simulink model "sixdof"  (R2023a)
settings: Solver=FixedStepAuto  StartTime=0.0  StopTime=5000  FixedStep=0.01  RelTol=1e-3  EnableMultiTasking=on
InitFcn:
  | fox_loadvariables_new
model workspace (MAT data in the model file):
  waypoints = [0  0  20; 1000  0  20; 1000  1000  20; -1000  1000  20; 0  0  20]
values from neighbouring files (symbols this model uses):
  Apolar = 0.038    [fox_loadvariables_new.m]
  CD0 = 0.0191    [fox_loadvariables_new.m]
  chord = chord*0.3048    (= 0.3048)    [fox_loadvariables_new.m]
  CL0 = 3*0.076    (= 0.228)    [fox_loadvariables_new.m]
  CLa = 5.097    [fox_loadvariables_new.m]
  CLa_dot = 1.93    [fox_loadvariables_new.m]
  Clb = -0.0598    [fox_loadvariables_new.m]
  ClDa = 0.265    [fox_loadvariables_new.m]
  CLDe = 0.738    [fox_loadvariables_new.m]
  ClDr = 0.0064    [fox_loadvariables_new.m]
  Clp = -0.363    [fox_loadvariables_new.m]
  CLq = 6.03    [fox_loadvariables_new.m]
  Clr = 0.0886    [fox_loadvariables_new.m]
  Cm0 = 0.107    [fox_loadvariables_new.m]
  Cma = -2.051    [fox_loadvariables_new.m]
  Cma_dot = -5.286    [fox_loadvariables_new.m]
  CmDe = -2.021    [fox_loadvariables_new.m]
  Cmq = -16.52    [fox_loadvariables_new.m]
  Cnb = 0.0562    [fox_loadvariables_new.m]
  CnDa = -0.0296    [fox_loadvariables_new.m]
  CnDr = -0.0377    [fox_loadvariables_new.m]
  Cnp = -0.0407    [fox_loadvariables_new.m]
  Cnr = -0.0439    [fox_loadvariables_new.m]
  CYb = -0.204    [fox_loadvariables_new.m]
  CYDr = 0.112    [fox_loadvariables_new.m]
  Euler_0 = [0; 0; 180]'*pi/180    [fox_loadvariables_new.m]
  ISA_g = 9.815    [fox_loadvariables_new.m]
  ISA_hmax = 2000    [fox_loadvariables_new.m]
  ISA_lapse = .0065    (= 0.0065)    [fox_loadvariables_new.m]
  ISA_P0 = 101325    [fox_loadvariables_new.m]
  ISA_R = 287    [fox_loadvariables_new.m]
  ISA_rho0 = 1.225    [fox_loadvariables_new.m]
  ISA_T0 = 289    [fox_loadvariables_new.m]
  Ixx = Ixx*1.355817949    (= 0.363359210332)    [fox_loadvariables_new.m]
  Iyy = Iyy*1.355817949    (= 0.86772348736)    [fox_loadvariables_new.m]
  Izz = Izz*1.355817949    (= 1.19854306692)    [fox_loadvariables_new.m]
  mass = mass*0.45359237    (= 9.0718474)    [fox_loadvariables_new.m]
  Pos_0 = [0; 0; 100.]    [fox_loadvariables_new.m]
  PQR_0 = [0; 0; 0]'    [fox_loadvariables_new.m]
  span = span*0.3048    (= 2.4384)    [fox_loadvariables_new.m]
  Vb_0 = [85.; 0; 0]'*0.3048    [fox_loadvariables_new.m]
undefined symbols (not defined in the file or in its folder): YPGwind
libraries: simulink x5, slpidlib x5, sharedtransform x1, uavutilslib x1, uavalgslib x1
(part 1 of 2)
settings Model: Creator=anouck  LastModifiedBy=terry
settings SolverCC: AlgebraicLoopSolver=TrustRegion  EnableFixedStepZeroCrossing=on
settings DataIOCC: LimitDataPoints=on  SaveFormat=Array  SignalLoggingSaveFormat=ModelDataLogs  ReturnWorkspaceOutputs=off  SignalLoggingName=sigsOut
settings OptimizationCC: ExpressionDepthLimit=2147483647  LifeSpan=inf
settings DebuggingCC: SaveWithParameterizedLinksMsg=none  UnderspecifiedInitializationDetection=Classic  MergeDetectMultiDrivingBlocksExec=none  SignalResolutionControl=TryResolveAllWithWarning  MultiTaskDSMMsg=warning  MultiTaskCondExecSysMsg=none  FcnCallInpInsideContextMsg=warning  UnconnectedInputMsg=warning  UnconnectedOutputMsg=warning  UnconnectedLineMsg=warning  StateNameClashWarn=warning  SFUnexpectedBacktrackingDiag=warning  SFNoUnconditionalDefaultTransitionDiag=warning  SFExecutionAtInitializationDiag=none  ArithmeticOperatorsInVariantConditions=warning
settings HardwareCC: ProdBitPerPointer=32  ProdBitPerSizeT=32  ProdBitPerPtrDiffT=32  ProdLargestAtomicFloat=None  ProdIntDivRoundTo=Undefined  ProdEndianess=Unspecified  ProdWordSize=32  ProdHWDeviceType=32-bit Generic  TargetBitPerPointer=64  TargetBitPerSizeT=64  TargetBitPerPtrDiffT=64  TargetLongLongMode=on  TargetIntDivRoundTo=Zero  TargetEndianess=LittleEndian  TargetWordSize=64  TargetHWDeviceType=MATLAB Host  ProdEqTarget=off
settings ModelReferenceCC: PropagateSignalLabelsOutOfModel=off
settings SFSimCC: SimUseLocalCustomCode=off  CustomCodeUndefinedFunction=UseInterfaceOnly
settings RTWCC: RTWUseLocalCustomCode=off
settings CodeAppCC: StateflowObjectComments=on
settings GRTTargetCC: TargetLangStandard=C89/C90 (ANSI)  CombineOutputUpdateFcns=off  GRTInterface=on
settings ConfigComp: CovMetricSettings=dw  CovSaveCumulativeToWorkspaceVar=on  CovSaveSingleToWorkspaceVar=on  CovExternalEMLEnable=off

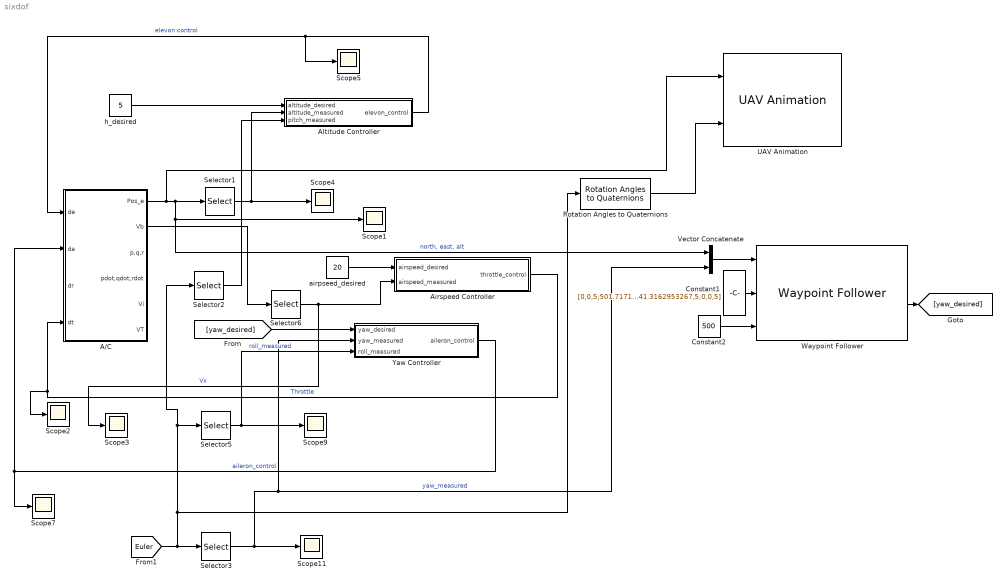
== system sixdof ==
  A/C : Subsystem
  Airspeed Controller : Subsystem
  Altitude Controller : Subsystem
  Constant1 : Constant  Value=[0,0,5;501.717105508643,908.922660414421,5;3007.34596928847,2458.44221262396,5;5143.8601437273,2189.82336415166,5;4248.4135386412,823.96084565673,5;2381.03201490461,241.3162953267,5;0,0,5]
  Constant2 : Constant  Value=500
  Rotation Angles to Quaternions : sharedtransform/Rotation Angles to Quaternions  rotationOrder=XYZ  aMode=aMode
  Scope{1..5,7,9,11} (8 alike) : Scope
  Selector1 : Selector  InputPortWidth=3  IndexOptions=Index vector (dialog)  Indices=3  OutputSizes=1
  Selector2 : Selector  InputPortWidth=3  IndexOptions=Index vector (dialog)  Indices=2  OutputSizes=1
  Selector3 : Selector  InputPortWidth=3  IndexOptions=Index vector (dialog)  Indices=3  OutputSizes=1
  Selector5 : Selector  InputPortWidth=3  IndexOptions=Index vector (dialog)  Indices=1  OutputSizes=1
  Selector6 : Selector  InputPortWidth=3  IndexOptions=Index vector (dialog)  Indices=1  OutputSizes=1
  UAV Animation : uavutilslib/UAV Animation  UAVType=FixedWing  UAVSize=100  InertialZDirection=Up  SampleTime=-1
  Vector Concatenate : Concatenate
  Waypoint Follower : uavalgslib/Waypoint Follower  UAVType=multirotor  StartFrom=first  TransitionRadiusSource=internal  TransitionRadius=10  MinLookaheadDistance=0.1  YawInput=off  ShowCrossTrackErrorOutput=off  ShowStatusOutput=off  SimulateUsing=Interpreted execution
  Yaw Controller : Subsystem
  airpseed_desired : Constant  Value=20
  h_desired : Constant  Value=5
  wires:
  A/C/1(Pos_e) -> UAV Animation/1, Scope1/1, Vector Concatenate/1, Selector1/1  "north, east, alt"
  Selector1/1 -> Altitude Controller/2(altitude_measured), Scope4/1
  h_desired/1 -> Altitude Controller/1(altitude_desired)
  Selector2/1 -> Altitude Controller/3(pitch_measured)
  Altitude Controller/1(elevon_control) -> A/C/1(de), Scope5/1  "elevon control"
  Selector5/1 -> Yaw Controller/3(roll_measured), Scope9/1  "roll_measured"
  Yaw Controller/1(aileron_control) -> A/C/2(da), Scope7/1  "aileron_control"
  Selector3/1 -> Yaw Controller/2(yaw_measured), Vector Concatenate/2, Scope11/1  "yaw_measured"
  Selector6/1 -> Airspeed Controller/2(airspeed_measured), Scope3/1  "Vx"
  airpseed_desired/1 -> Airspeed Controller/1(airspeed_desired)
  Airspeed Controller/1(throttle_control) -> A/C/4(dt), Scope2/1  "Throttle"
  Rotation Angles to Quaternions/1 -> UAV Animation/2
  Waypoint Follower/3 -> [yaw_desired]
  [Euler] -> Rotation Angles to Quaternions/1, Selector2/1, Selector5/1, Selector3/1
  Vector Concatenate/1 -> Waypoint Follower/1
  Constant2/1 -> Waypoint Follower/3
  A/C/2(Vb) -> Selector6/1
  Constant1/1 -> Waypoint Follower/2
  [yaw_desired] -> Yaw Controller/1(yaw_desired)

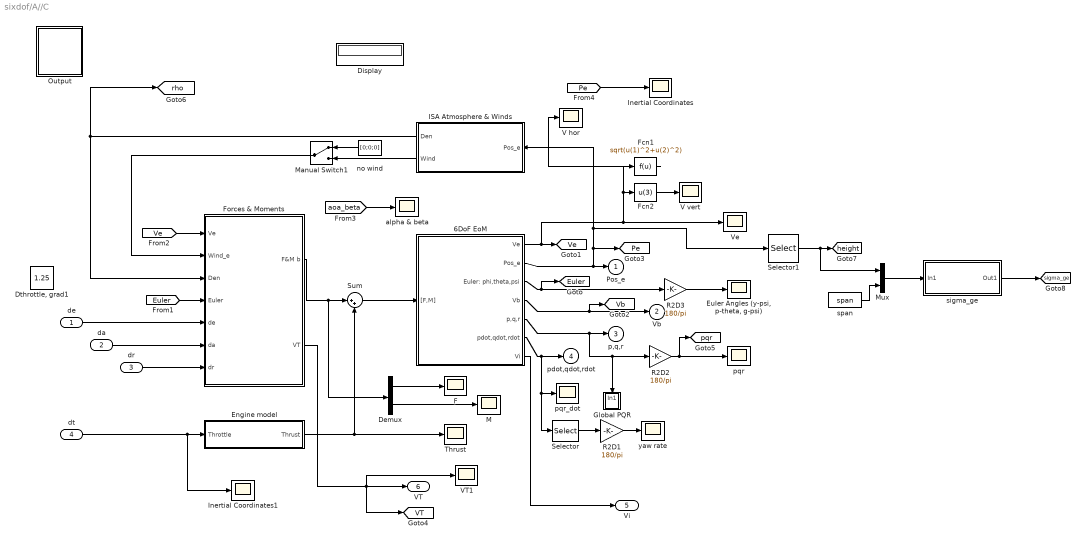
== system sixdof/A//C ==
  de : Inport
  da : Inport  Port=2
  dr : Inport  Port=3
  dt : Inport  Port=4
  " no wind" : Constant  Value=[0;0;0]  VectorParams1D=off
  6DoF EoM : Subsystem
  Demux : Demux  Outputs=2
      settings: DisplayOption=none
  Display : Display
  "Dthrottle, grad1" : Constant  Value=1.25
  Engine model : Subsystem
  "Euler Angles (y-psi, p-theta, g-psi)" : Scope
  F : Scope
  Fcn1 : Fcn  Expr=sqrt(u(1)^2+u(2)^2)
  Fcn2 : Fcn  Expr=u(3)
  Forces & Moments : Subsystem
  Global PQR : Subsystem
  ISA Atmosphere & Winds : Subsystem
  Inertial Coordinates : Scope
  Inertial Coordinates1 : Scope
  M : Scope
  Manual Switch1 : ManualSwitch
  Mux : Mux  Inputs=2
  Output : Subsystem
  R2D1 : Gain  Gain=180/pi  SaturateOnIntegerOverflow=on  OutDataTypeStr=Inherit: Same as input  ParamDataTypeStr=Inherit: Same as input
  R2D2 : Gain  Gain=180/pi  SaturateOnIntegerOverflow=on  OutDataTypeStr=Inherit: Same as input  ParamDataTypeStr=Inherit: Same as input
  R2D3 : Gain  Gain=180/pi  SaturateOnIntegerOverflow=on  OutDataTypeStr=Inherit: Same as input  ParamDataTypeStr=Inherit: Same as input
  Selector : Selector  InputPortWidth=3  IndexOptions=Index vector (dialog)  Indices=3  OutputSizes=1
  Selector1 : Selector  InputPortWidth=3  IndexOptions=Index vector (dialog)  Indices=[3]  OutputSizes=1
  Sum : Sum  Inputs=|++  SaturateOnIntegerOverflow=on
  Thrust : Scope
  V hor : Scope
  V vert : Scope
  VT1 : Scope
  Ve : Scope
  alpha & beta : Scope
  pqr : Scope
  pqr_dot : Scope
  sigma_ge : Subsystem
  span : Constant  Value=span  VectorParams1D=off
  yaw rate : Scope
  Pos_e : Outport  InitialOutput=0
  Vb : Outport  Port=2  InitialOutput=0
  p,q,r : Outport  Port=3  InitialOutput=0
  pdot,qdot,rdot : Outport  Port=4  InitialOutput=0
  Vi : Outport  Port=5
  VT : Outport  Port=6
  tag scope: Euler=global, Pe=global, VT=global, Vb=global, Ve=global, height=global, pqr=global, rho=global, sigma_ge=global
  wires:
  6DoF EoM/1(Ve) -> [Ve], Ve/1, Fcn2/1, Fcn1/1
  6DoF EoM/4(Vb) -> [Vb], Vb/1
  6DoF EoM/3(Euler: phi,theta,psi) -> R2D3/1, [Euler]
  6DoF EoM/6(pdot,qdot,rdot) -> pqr_dot/1, Selector/1, pdot,qdot,rdot/1
  6DoF EoM/5(p,q,r) -> p,q,r/1, Global PQR/1(In1), R2D2/1
  Demux/1 -> F/1
  [Euler] -> Forces & Moments/4(Euler)
  [Ve] -> Forces & Moments/1(Ve)
  R2D3/1 -> "Euler Angles (y-psi, p-theta, g-psi)"/1
  ISA Atmosphere & Winds/2(Wind) -> Manual Switch1/2
  " no wind"/1 -> Manual Switch1/1
  R2D2/1 -> pqr/1, [pqr]
  [Pe] -> Inertial Coordinates/1
  Manual Switch1/1 -> Forces & Moments/2(Wind_e)
  Fcn1/1 -> V hor/1
  R2D1/1 -> yaw rate/1
  Demux/2 -> M/1
  Sum/1 -> 6DoF EoM/1("[F,M]")
  Forces & Moments/1(F&M b) -> Sum/1, Demux/1
  Engine model/1(Thrust) -> Thrust/1, Sum/2
  [aoa_beta] -> alpha & beta/1
  Fcn2/1 -> V vert/1
  Selector/1 -> R2D1/1
  de/1 -> Forces & Moments/5(de)
  da/1 -> Forces & Moments/6(da)
  dr/1 -> Forces & Moments/7(dr)
  6DoF EoM/7(Vi) -> Vi/1
  dt/1 -> Engine model/1(Throttle), Inertial Coordinates1/1
  Forces & Moments/2(VT) -> VT/1, [VT], VT1/1
  ISA Atmosphere & Winds/1(Den) -> Forces & Moments/3(Den), [rho]
  6DoF EoM/2(Pos_e) -> Pos_e/1, Selector1/1, ISA Atmosphere & Winds/1(Pos_e), [Pe]
  Selector1/1 -> Mux/1, [height]
  span/1 -> Mux/2
  Mux/1 -> sigma_ge/1(In1)
  sigma_ge/1(Out1) -> [sigma_ge]

== system sixdof/Airspeed Controller ==
  airspeed_desired : Inport
  airspeed_measured : Inport  Port=2
  Discrete PID Controller4 : slpidlib/PID Controller  Controller=PID  Form=Parallel  TimeDomain=Discrete-time  UseExternalTs=off  SampleTime=-1  IntegratorMethod=Forward Euler  FilterMethod=Forward Euler  ControllerParametersSource=internal  P=.7  I=0.0145240090706121  UseKiTs=off  D=0  N=0  UseFilter=off  TunerSelectOption=Frequency Response Based  InitialConditionSource=internal  InitialConditionForIntegrator=0  InitialConditionForFilter=0  DifferentiatorICPrevScaledInput=0  ExternalReset=none  TrackingMode=off  Kt=1  LimitOutput=on  SatLimitsSource=internal  UpperSaturationLimit=2  LowerSaturationLimit=0  LinearizeAsGain=off  AntiWindupMode=none  Kb=1  LimitIntegrator=off  UpperIntegratorSaturationLimit=inf  LowerIntegratorSaturationLimit=-inf  POutMin=[]  POutMax=[]  IOutMin=[]  IOutMax=[]  DOutMin=[]  DOutMax=[]  NOutMin=[]  NOutMax=[]  SumOutMin=[]  SumOutMax=[]  SaturationOutMin=[]  SaturationOutMax=[]  PParamMin=[]  PParamMax=[]  IParamMin=[]  IParamMax=[]  DParamMin=[]  DParamMax=[]  NParamMin=[]  NParamMax=[]  KbParamMin=[]  KbParamMax=[]  KtParamMin=[]  KtParamMax=[]  KbOutMin=[]  KbOutMax=[]  KtOutMin=[]  KtOutMax=[]  IntegratorOutMin=[]  IntegratorOutMax=[]  FilterOutMin=[]  FilterOutMax=[]  SumI1OutMin=[]  SumI1OutMax=[]  SumI2OutMin=[]  SumI2OutMax=[]  SumI3OutMin=[]  SumI3OutMax=[]  SumI4OutMin=[]  SumI4OutMax=[]  SumDOutMin=[]  SumDOutMax=[]  DifferentiatorOutMin=[]  DifferentiatorOutMax=[]  FilterDiffOutCoefMin=[]  FilterDiffOutCoefMax=[]  ReciprocalOutMin=[]  ReciprocalOutMax=[]  SumDenOutMin=[]  SumDenOutMax=[]  SumNumOutMin=[]  SumNumOutMax=[]  DivideOutMin=[]  DivideOutMax=[]  UdiffTsProdOutMin=[]  UdiffTsProdOutMax=[]  NTsProdOutMin=[]  NTsProdOutMax=[]  UintegralTsProdOutMin=[]  UintegralTsProdOutMax=[]  UngainTsProdOutMin=[]  UngainTsProdOutMax=[]  ClampingZeroOutDataTypeStr=Inherit: Inherit via back propagation  ClampingZeroOutMin=[]  ClampingZeroOutMax=[]  FilterDenConstantOutDataTypeStr=Inherit: Inherit via back propagation  FilterDenConstantOutMin=[]  FilterDenConstantOutMax=[]  PCopyOutDataTypeStr=Inherit: Inherit via back propagation  PCopyOutMin=[]  PCopyOutMax=[]  NCopyOutDataTypeStr=Inherit: Inherit via back propagation  NCopyOutMin=[]  NCopyOutMax=[]  IntegratorContinuousStateAttributes=''  IntegratorStateMustResolveToSignalObject=off  IntegratorRTWStateStorageClass=Auto  FilterContinuousStateAttributes=''  FilterStateMustResolveToSignalObject=off  FilterRTWStateStorageClass=Auto  ParallelPVariant=InternalParameters  IdealPVariant=Disabled  IVariant=InternalParameters  DVariant=InternalParameters  IntegratorVariant=Discrete  SatVariant=Enabled  AWVariant=Passthrough  PCopyVariant=Disabled  TRVariant=Disabled  FdbkBlocksVariant=Forward  IdealPFdbkVariant=Disabled  SatFdbkVariant=Disabled  DerivativeFilterVariant=Differentiator  NVariant=Passthrough  NCopyVariant=Disabled_SignalSpec  FilterICVariant=InternalICsDifferentiator  IntegratorICVariant=InternalICs  ExternalResetVariant=Disabled  TRSumVariant=Passthrough  SumFdbkVariant=Disabled  SumVariant=Sum_PID  TsampFilterVariant=InternalTs  TsampNgainVariant=Passthrough  TsampIntegralVariant=Disabled_SignalSpec  ExternalSaturationOutDataTypeStr=Inherit: Same as second input
      settings: LibrarySourceBlock=simulink/Discrete/Discrete PID Controller
  Subtract4 : Sum  Inputs=+-
  throttle_control : Outport
  wires:
  Subtract4/1 -> Discrete PID Controller4/1  "airspeed_error"
  airspeed_desired/1 -> Subtract4/1
  airspeed_measured/1 -> Subtract4/2
  Discrete PID Controller4/1 -> throttle_control/1  "Throttle"

== system sixdof/Altitude Controller ==
  altitude_desired : Inport
  altitude_measured : Inport  Port=2
  pitch_measured : Inport  Port=3
  Discrete PID Controller : slpidlib/PID Controller  Controller=PID  Form=Parallel  TimeDomain=Discrete-time  UseExternalTs=off  SampleTime=-1  IntegratorMethod=Forward Euler  FilterMethod=Forward Euler  ControllerParametersSource=internal  P=-0.5  I=0  UseKiTs=off  D=0  N=100  UseFilter=off  TunerSelectOption=Transfer Function Based (PID Tuner App)  InitialConditionSource=internal  InitialConditionForIntegrator=0  InitialConditionForFilter=0  DifferentiatorICPrevScaledInput=0  ExternalReset=none  TrackingMode=off  Kt=1  LimitOutput=off  SatLimitsSource=internal  UpperSaturationLimit=inf  LowerSaturationLimit=-inf  LinearizeAsGain=off  AntiWindupMode=none  Kb=1  LimitIntegrator=off  UpperIntegratorSaturationLimit=inf  LowerIntegratorSaturationLimit=-inf  POutMin=[]  POutMax=[]  IOutMin=[]  IOutMax=[]  DOutMin=[]  DOutMax=[]  NOutMin=[]  NOutMax=[]  SumOutMin=[]  SumOutMax=[]  SaturationOutMin=[]  SaturationOutMax=[]  PParamMin=[]  PParamMax=[]  IParamMin=[]  IParamMax=[]  DParamMin=[]  DParamMax=[]  NParamMin=[]  NParamMax=[]  KbParamMin=[]  KbParamMax=[]  KtParamMin=[]  KtParamMax=[]  KbOutMin=[]  KbOutMax=[]  KtOutMin=[]  KtOutMax=[]  IntegratorOutMin=[]  IntegratorOutMax=[]  FilterOutMin=[]  FilterOutMax=[]  SumI1OutMin=[]  SumI1OutMax=[]  SumI2OutMin=[]  SumI2OutMax=[]  SumI3OutMin=[]  SumI3OutMax=[]  SumI4OutMin=[]  SumI4OutMax=[]  SumDOutMin=[]  SumDOutMax=[]  DifferentiatorOutMin=[]  DifferentiatorOutMax=[]  FilterDiffOutCoefMin=[]  FilterDiffOutCoefMax=[]  ReciprocalOutMin=[]  ReciprocalOutMax=[]  SumDenOutMin=[]  SumDenOutMax=[]  SumNumOutMin=[]  SumNumOutMax=[]  DivideOutMin=[]  DivideOutMax=[]  UdiffTsProdOutMin=[]  UdiffTsProdOutMax=[]  NTsProdOutMin=[]  NTsProdOutMax=[]  UintegralTsProdOutMin=[]  UintegralTsProdOutMax=[]  UngainTsProdOutMin=[]  UngainTsProdOutMax=[]  ClampingZeroOutDataTypeStr=Inherit: Inherit via back propagation  ClampingZeroOutMin=[]  ClampingZeroOutMax=[]  FilterDenConstantOutDataTypeStr=Inherit: Inherit via back propagation  FilterDenConstantOutMin=[]  FilterDenConstantOutMax=[]  PCopyOutDataTypeStr=Inherit: Inherit via back propagation  PCopyOutMin=[]  PCopyOutMax=[]  NCopyOutDataTypeStr=Inherit: Inherit via back propagation  NCopyOutMin=[]  NCopyOutMax=[]  IntegratorContinuousStateAttributes=''  IntegratorStateMustResolveToSignalObject=off  IntegratorRTWStateStorageClass=Auto  FilterContinuousStateAttributes=''  FilterStateMustResolveToSignalObject=off  FilterRTWStateStorageClass=Auto  ParallelPVariant=InternalParameters  IdealPVariant=Disabled  IVariant=InternalParameters  DVariant=InternalParameters  IntegratorVariant=Discrete  SatVariant=Disabled  AWVariant=Passthrough  PCopyVariant=Disabled  TRVariant=Disabled  FdbkBlocksVariant=Forward  IdealPFdbkVariant=Disabled  SatFdbkVariant=Disabled  DerivativeFilterVariant=Differentiator  NVariant=Passthrough  NCopyVariant=Disabled_SignalSpec  FilterICVariant=InternalICsDifferentiator  IntegratorICVariant=InternalICs  ExternalResetVariant=Disabled  TRSumVariant=Passthrough  SumFdbkVariant=Disabled  SumVariant=Sum_PID  TsampFilterVariant=InternalTs  TsampNgainVariant=Passthrough  TsampIntegralVariant=Disabled_SignalSpec  ExternalSaturationOutDataTypeStr=Inherit: Same as second input
      settings: LibrarySourceBlock=simulink/Discrete/Discrete PID Controller
  Discrete PID Controller1 : slpidlib/PID Controller  Controller=PID  Form=Parallel  TimeDomain=Discrete-time  UseExternalTs=off  SampleTime=-1  IntegratorMethod=Forward Euler  FilterMethod=Forward Euler  ControllerParametersSource=internal  P=.8  I=.01  UseKiTs=off  D=.5  N=100  UseFilter=off  TunerSelectOption=Transfer Function Based (PID Tuner App)  InitialConditionSource=internal  InitialConditionForIntegrator=0  InitialConditionForFilter=0  DifferentiatorICPrevScaledInput=0  ExternalReset=none  TrackingMode=off  Kt=1  LimitOutput=on  SatLimitsSource=internal  UpperSaturationLimit=5  LowerSaturationLimit=-2  LinearizeAsGain=off  AntiWindupMode=none  Kb=1  LimitIntegrator=off  UpperIntegratorSaturationLimit=inf  LowerIntegratorSaturationLimit=-inf  POutMin=[]  POutMax=[]  IOutMin=[]  IOutMax=[]  DOutMin=[]  DOutMax=[]  NOutMin=[]  NOutMax=[]  SumOutMin=[]  SumOutMax=[]  SaturationOutMin=[]  SaturationOutMax=[]  PParamMin=[]  PParamMax=[]  IParamMin=[]  IParamMax=[]  DParamMin=[]  DParamMax=[]  NParamMin=[]  NParamMax=[]  KbParamMin=[]  KbParamMax=[]  KtParamMin=[]  KtParamMax=[]  KbOutMin=[]  KbOutMax=[]  KtOutMin=[]  KtOutMax=[]  IntegratorOutMin=[]  IntegratorOutMax=[]  FilterOutMin=[]  FilterOutMax=[]  SumI1OutMin=[]  SumI1OutMax=[]  SumI2OutMin=[]  SumI2OutMax=[]  SumI3OutMin=[]  SumI3OutMax=[]  SumI4OutMin=[]  SumI4OutMax=[]  SumDOutMin=[]  SumDOutMax=[]  DifferentiatorOutMin=[]  DifferentiatorOutMax=[]  FilterDiffOutCoefMin=[]  FilterDiffOutCoefMax=[]  ReciprocalOutMin=[]  ReciprocalOutMax=[]  SumDenOutMin=[]  SumDenOutMax=[]  SumNumOutMin=[]  SumNumOutMax=[]  DivideOutMin=[]  DivideOutMax=[]  UdiffTsProdOutMin=[]  UdiffTsProdOutMax=[]  NTsProdOutMin=[]  NTsProdOutMax=[]  UintegralTsProdOutMin=[]  UintegralTsProdOutMax=[]  UngainTsProdOutMin=[]  UngainTsProdOutMax=[]  ClampingZeroOutDataTypeStr=Inherit: Inherit via back propagation  ClampingZeroOutMin=[]  ClampingZeroOutMax=[]  FilterDenConstantOutDataTypeStr=Inherit: Inherit via back propagation  FilterDenConstantOutMin=[]  FilterDenConstantOutMax=[]  PCopyOutDataTypeStr=Inherit: Inherit via back propagation  PCopyOutMin=[]  PCopyOutMax=[]  NCopyOutDataTypeStr=Inherit: Inherit via back propagation  NCopyOutMin=[]  NCopyOutMax=[]  IntegratorContinuousStateAttributes=''  IntegratorStateMustResolveToSignalObject=off  IntegratorRTWStateStorageClass=Auto  FilterContinuousStateAttributes=''  FilterStateMustResolveToSignalObject=off  FilterRTWStateStorageClass=Auto  ParallelPVariant=InternalParameters  IdealPVariant=Disabled  IVariant=InternalParameters  DVariant=InternalParameters  IntegratorVariant=Discrete  SatVariant=Enabled  AWVariant=Passthrough  PCopyVariant=Disabled  TRVariant=Disabled  FdbkBlocksVariant=Forward  IdealPFdbkVariant=Disabled  SatFdbkVariant=Disabled  DerivativeFilterVariant=Differentiator  NVariant=Passthrough  NCopyVariant=Disabled_SignalSpec  FilterICVariant=InternalICsDifferentiator  IntegratorICVariant=InternalICs  ExternalResetVariant=Disabled  TRSumVariant=Passthrough  SumFdbkVariant=Disabled  SumVariant=Sum_PID  TsampFilterVariant=InternalTs  TsampNgainVariant=Passthrough  TsampIntegralVariant=Disabled_SignalSpec  ExternalSaturationOutDataTypeStr=Inherit: Same as second input
      settings: LibrarySourceBlock=simulink/Discrete/Discrete PID Controller
  Subtract : Sum  Inputs=+-
  Subtract1 : Sum  Inputs=+-
  elevon_control : Outport
  wires:
  Subtract1/1 -> Discrete PID Controller1/1  "pitch_error"
  Subtract/1 -> Discrete PID Controller/1  "altitude_error"
  Discrete PID Controller/1 -> Subtract1/1  "pitch_desired"
  altitude_measured/1 -> Subtract/2
  altitude_desired/1 -> Subtract/1
  Discrete PID Controller1/1 -> elevon_control/1  "elevon control"
  pitch_measured/1 -> Subtract1/2

== system sixdof/Yaw Controller ==
  yaw_desired : Inport
  yaw_measured : Inport  Port=2
  roll_measured : Inport  Port=3
  Discrete PID Controller2 : slpidlib/PID Controller  Controller=PID  Form=Parallel  TimeDomain=Discrete-time  UseExternalTs=off  SampleTime=-1  IntegratorMethod=Forward Euler  FilterMethod=Forward Euler  ControllerParametersSource=internal  P=0.5  I=0  UseKiTs=off  D=0  N=100  UseFilter=on  TunerSelectOption=Transfer Function Based (PID Tuner App)  InitialConditionSource=internal  InitialConditionForIntegrator=0  InitialConditionForFilter=0  DifferentiatorICPrevScaledInput=0  ExternalReset=none  TrackingMode=off  Kt=1  LimitOutput=off  SatLimitsSource=internal  UpperSaturationLimit=inf  LowerSaturationLimit=-inf  LinearizeAsGain=off  AntiWindupMode=none  Kb=1  LimitIntegrator=off  UpperIntegratorSaturationLimit=inf  LowerIntegratorSaturationLimit=-inf  POutMin=[]  POutMax=[]  IOutMin=[]  IOutMax=[]  DOutMin=[]  DOutMax=[]  NOutMin=[]  NOutMax=[]  SumOutMin=[]  SumOutMax=[]  SaturationOutMin=[]  SaturationOutMax=[]  PParamMin=[]  PParamMax=[]  IParamMin=[]  IParamMax=[]  DParamMin=[]  DParamMax=[]  NParamMin=[]  NParamMax=[]  KbParamMin=[]  KbParamMax=[]  KtParamMin=[]  KtParamMax=[]  KbOutMin=[]  KbOutMax=[]  KtOutMin=[]  KtOutMax=[]  IntegratorOutMin=[]  IntegratorOutMax=[]  FilterOutMin=[]  FilterOutMax=[]  SumI1OutMin=[]  SumI1OutMax=[]  SumI2OutMin=[]  SumI2OutMax=[]  SumI3OutMin=[]  SumI3OutMax=[]  SumI4OutMin=[]  SumI4OutMax=[]  SumDOutMin=[]  SumDOutMax=[]  DifferentiatorOutMin=[]  DifferentiatorOutMax=[]  FilterDiffOutCoefMin=[]  FilterDiffOutCoefMax=[]  ReciprocalOutMin=[]  ReciprocalOutMax=[]  SumDenOutMin=[]  SumDenOutMax=[]  SumNumOutMin=[]  SumNumOutMax=[]  DivideOutMin=[]  DivideOutMax=[]  UdiffTsProdOutMin=[]  UdiffTsProdOutMax=[]  NTsProdOutMin=[]  NTsProdOutMax=[]  UintegralTsProdOutMin=[]  UintegralTsProdOutMax=[]  UngainTsProdOutMin=[]  UngainTsProdOutMax=[]  ClampingZeroOutDataTypeStr=Inherit: Inherit via back propagation  ClampingZeroOutMin=[]  ClampingZeroOutMax=[]  FilterDenConstantOutDataTypeStr=Inherit: Inherit via back propagation  FilterDenConstantOutMin=[]  FilterDenConstantOutMax=[]  PCopyOutDataTypeStr=Inherit: Inherit via back propagation  PCopyOutMin=[]  PCopyOutMax=[]  NCopyOutDataTypeStr=Inherit: Inherit via back propagation  NCopyOutMin=[]  NCopyOutMax=[]  IntegratorContinuousStateAttributes=''  IntegratorStateMustResolveToSignalObject=off  IntegratorRTWStateStorageClass=Auto  FilterContinuousStateAttributes=''  FilterStateMustResolveToSignalObject=off  FilterRTWStateStorageClass=Auto  ParallelPVariant=InternalParameters  IdealPVariant=Disabled  IVariant=InternalParameters  DVariant=InternalParameters  IntegratorVariant=Discrete  SatVariant=Disabled  AWVariant=Passthrough  PCopyVariant=Disabled  TRVariant=Disabled  FdbkBlocksVariant=Forward  IdealPFdbkVariant=Disabled  SatFdbkVariant=Disabled  DerivativeFilterVariant=ForwardEulerFilter  NVariant=InternalParameters  NCopyVariant=Disabled  FilterICVariant=InternalICsFilter  IntegratorICVariant=InternalICs  ExternalResetVariant=Disabled  TRSumVariant=Passthrough  SumFdbkVariant=Disabled  SumVariant=Sum_PID  TsampFilterVariant=InternalTs  TsampNgainVariant=Passthrough  TsampIntegralVariant=Disabled_SignalSpec  ExternalSaturationOutDataTypeStr=Inherit: Same as second input
      settings: LibrarySourceBlock=simulink/Discrete/Discrete PID Controller
  Discrete PID Controller3 : slpidlib/PID Controller  Controller=PID  Form=Parallel  TimeDomain=Discrete-time  UseExternalTs=off  SampleTime=-1  IntegratorMethod=Forward Euler  FilterMethod=Forward Euler  ControllerParametersSource=internal  P=.5  I=0  UseKiTs=off  D=5  N=100  UseFilter=on  TunerSelectOption=Transfer Function Based (PID Tuner App)  InitialConditionSource=internal  InitialConditionForIntegrator=0  InitialConditionForFilter=0  DifferentiatorICPrevScaledInput=0  ExternalReset=none  TrackingMode=off  Kt=1  LimitOutput=on  SatLimitsSource=internal  UpperSaturationLimit=1  LowerSaturationLimit=-1  LinearizeAsGain=off  AntiWindupMode=none  Kb=1  LimitIntegrator=off  UpperIntegratorSaturationLimit=inf  LowerIntegratorSaturationLimit=-inf  POutMin=[]  POutMax=[]  IOutMin=[]  IOutMax=[]  DOutMin=[]  DOutMax=[]  NOutMin=[]  NOutMax=[]  SumOutMin=[]  SumOutMax=[]  SaturationOutMin=[]  SaturationOutMax=[]  PParamMin=[]  PParamMax=[]  IParamMin=[]  IParamMax=[]  DParamMin=[]  DParamMax=[]  NParamMin=[]  NParamMax=[]  KbParamMin=[]  KbParamMax=[]  KtParamMin=[]  KtParamMax=[]  KbOutMin=[]  KbOutMax=[]  KtOutMin=[]  KtOutMax=[]  IntegratorOutMin=[]  IntegratorOutMax=[]  FilterOutMin=[]  FilterOutMax=[]  SumI1OutMin=[]  SumI1OutMax=[]  SumI2OutMin=[]  SumI2OutMax=[]  SumI3OutMin=[]  SumI3OutMax=[]  SumI4OutMin=[]  SumI4OutMax=[]  SumDOutMin=[]  SumDOutMax=[]  DifferentiatorOutMin=[]  DifferentiatorOutMax=[]  FilterDiffOutCoefMin=[]  FilterDiffOutCoefMax=[]  ReciprocalOutMin=[]  ReciprocalOutMax=[]  SumDenOutMin=[]  SumDenOutMax=[]  SumNumOutMin=[]  SumNumOutMax=[]  DivideOutMin=[]  DivideOutMax=[]  UdiffTsProdOutMin=[]  UdiffTsProdOutMax=[]  NTsProdOutMin=[]  NTsProdOutMax=[]  UintegralTsProdOutMin=[]  UintegralTsProdOutMax=[]  UngainTsProdOutMin=[]  UngainTsProdOutMax=[]  ClampingZeroOutDataTypeStr=Inherit: Inherit via back propagation  ClampingZeroOutMin=[]  ClampingZeroOutMax=[]  FilterDenConstantOutDataTypeStr=Inherit: Inherit via back propagation  FilterDenConstantOutMin=[]  FilterDenConstantOutMax=[]  PCopyOutDataTypeStr=Inherit: Inherit via back propagation  PCopyOutMin=[]  PCopyOutMax=[]  NCopyOutDataTypeStr=Inherit: Inherit via back propagation  NCopyOutMin=[]  NCopyOutMax=[]  IntegratorContinuousStateAttributes=''  IntegratorStateMustResolveToSignalObject=off  IntegratorRTWStateStorageClass=Auto  FilterContinuousStateAttributes=''  FilterStateMustResolveToSignalObject=off  FilterRTWStateStorageClass=Auto  ParallelPVariant=InternalParameters  IdealPVariant=Disabled  IVariant=InternalParameters  DVariant=InternalParameters  IntegratorVariant=Discrete  SatVariant=Enabled  AWVariant=Passthrough  PCopyVariant=Disabled  TRVariant=Disabled  FdbkBlocksVariant=Forward  IdealPFdbkVariant=Disabled  SatFdbkVariant=Disabled  DerivativeFilterVariant=ForwardEulerFilter  NVariant=InternalParameters  NCopyVariant=Disabled  FilterICVariant=InternalICsFilter  IntegratorICVariant=InternalICs  ExternalResetVariant=Disabled  TRSumVariant=Passthrough  SumFdbkVariant=Disabled  SumVariant=Sum_PID  TsampFilterVariant=InternalTs  TsampNgainVariant=Passthrough  TsampIntegralVariant=Disabled_SignalSpec  ExternalSaturationOutDataTypeStr=Inherit: Same as second input
      settings: LibrarySourceBlock=simulink/Discrete/Discrete PID Controller
  Subtract2 : Sum  Inputs=+-
  Subtract3 : Sum  Inputs=+-
  aileron_control : Outport
  wires:
  Subtract2/1 -> Discrete PID Controller2/1  "yaw_error"
  Discrete PID Controller2/1 -> Subtract3/1  "roll_desired"
  roll_measured/1 -> Subtract3/2  "roll_measured"
  Subtract3/1 -> Discrete PID Controller3/1  "roll_error"
  yaw_desired/1 -> Subtract2/1
  yaw_measured/1 -> Subtract2/2  "yaw_mesured"
  Discrete PID Controller3/1 -> aileron_control/1  "aileron_control"

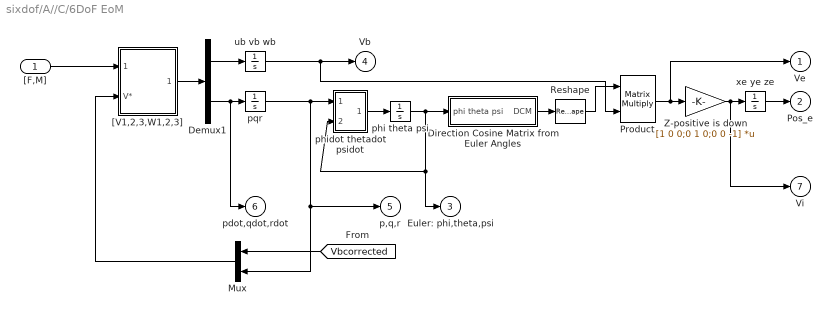
== system sixdof/A//C/6DoF EoM ==
  "[F,M]" : Inport
  Demux1 : Demux  Outputs=2
  Direction Cosine Matrix from Euler Angles : Subsystem
  Mux : Mux  Inputs=[3;3]
  Product : Product  Multiplication=Matrix(*)  InputSameDT=on  SaturateOnIntegerOverflow=on  OutDataTypeStr=Inherit: Same as first input
  Reshape : Reshape  OutputDimensionality=Customize  OutputDimensions=[3,3]
  Z-positive is down : Gain  Gain=[1 0 0;0 1 0;0 0 -1]  Multiplication=Matrix(K*u)  SaturateOnIntegerOverflow=on  OutDataTypeStr=Inherit: Same as input  ParamDataTypeStr=Inherit: Same as input
  "[V1,2,3,W1,2,3]" : Subsystem
  phi theta psi : Integrator  InitialCondition=Euler_0
  phidot thetadot psidot : Subsystem
  pqr : Integrator  InitialCondition=PQR_0'
  ub vb wb : Integrator  InitialCondition=Vb_0'
  xe ye ze : Integrator  InitialCondition=Pos_0
  Ve : Outport  InitialOutput=0
  Pos_e : Outport  Port=2  InitialOutput=0
  Euler: phi,theta,psi : Outport  Port=3  InitialOutput=0
  Vb : Outport  Port=4  InitialOutput=0
  p,q,r : Outport  Port=5  InitialOutput=0
  pdot,qdot,rdot : Outport  Port=6  InitialOutput=0
  Vi : Outport  Port=7  InitialOutput=0
  wires:
  phi theta psi/1 -> phidot thetadot psidot/2(phi theta psi), Euler: phi,theta,psi/1, Direction Cosine Matrix from Euler Angles/1(phi theta psi)
  phidot thetadot psidot/1(phidot thetadot psidot) -> phi theta psi/1
  Direction Cosine Matrix from Euler Angles/1(DCM) -> Reshape/1
  Demux1/1 -> ub vb wb/1
  "[V1,2,3,W1,2,3]"/1(V*dot) -> Demux1/1
  Demux1/2 -> pqr/1, pdot,qdot,rdot/1
  "[F,M]"/1 -> "[V1,2,3,W1,2,3]"/1("[F ; M]")
  Reshape/1 -> Product/1
  ub vb wb/1 -> Vb/1, Product/2
  Product/1 -> Z-positive is down/1, Ve/1
  Mux/1 -> "[V1,2,3,W1,2,3]"/2(V*)
  Z-positive is down/1 -> xe ye ze/1, Vi/1
  xe ye ze/1 -> Pos_e/1
  pqr/1 -> phidot thetadot psidot/1(p q r), p,q,r/1, Mux/2
  [Vbcorrected] -> Mux/1

== system sixdof/A//C/Engine model ==
  Throttle : Inport
  Constant4 : Constant  Value=0
  Mux : Mux  Inputs=2
  Mux1 : Mux  Inputs=6
  Saturation : Saturate  UpperLimit=inf  LowerLimit=.1
  Saturation1 : Saturate  UpperLimit=inf  LowerLimit=1
  Static Thrust (lbs) : Fcn  Expr=-4.088+0.00146*u
  Throttle2RPM : Gain  Gain=9000  SaturateOnIntegerOverflow=on  OutDataTypeStr=Inherit: Same as input  ParamDataTypeStr=Inherit: Same as input
  Thrust (lbs) : Fcn  Expr=u(1)-0.0238*u(2)*sqrt(u(1))
  kg2N : Gain  Gain=ISA_g  SaturateOnIntegerOverflow=on  OutDataTypeStr=Inherit: Same as input  ParamDataTypeStr=Inherit: Same as input
  lbs2kg : Gain  Gain=0.45359237  SaturateOnIntegerOverflow=on  OutDataTypeStr=Inherit: Same as input  ParamDataTypeStr=Inherit: Same as input
  mps2fps : Gain  Gain=3.280839895  SaturateOnIntegerOverflow=on  OutDataTypeStr=Inherit: Same as input  ParamDataTypeStr=Inherit: Same as input
  Thrust : Outport
  wires:
  Throttle/1 -> Throttle2RPM/1
  Throttle2RPM/1 -> Static Thrust (lbs)/1
  Static Thrust (lbs)/1 -> Mux/1
  Mux/1 -> Saturation/1
  Thrust (lbs)/1 -> lbs2kg/1
  mps2fps/1 -> Mux/2
  [magV] -> mps2fps/1
  Mux1/1 -> Thrust/1
  lbs2kg/1 -> kg2N/1
  Constant4/1 -> Mux1/6, Mux1/2, Mux1/3, Mux1/4, Mux1/5
  kg2N/1 -> Saturation1/1
  Saturation/1 -> Thrust (lbs)/1
  Saturation1/1 -> Mux1/1

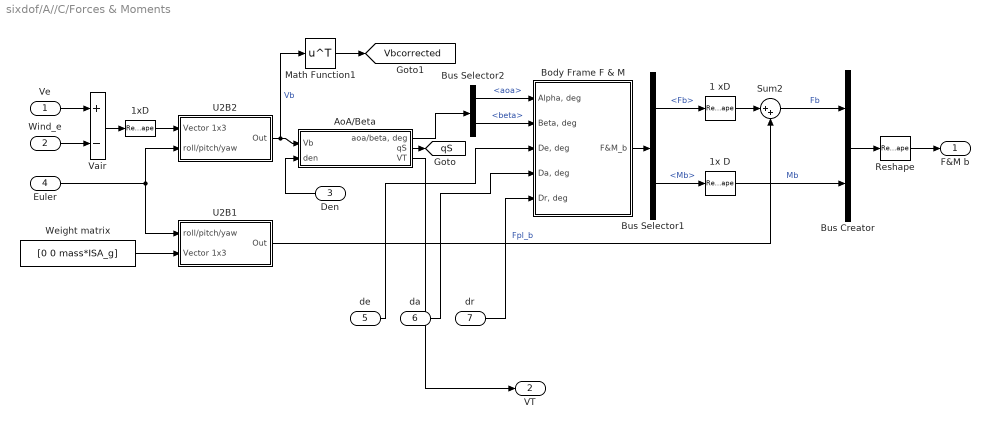
== system sixdof/A//C/Forces & Moments ==
  Ve : Inport
  Wind_e : Inport  Port=2
  Den : Inport  Port=3
  Euler : Inport  Port=4
  de : Inport  Port=5
  da : Inport  Port=6
  dr : Inport  Port=7
  1 xD : Reshape  OutputDimensionality=Row vector (2-D)
  1x D : Reshape  OutputDimensionality=Row vector (2-D)
  1xD : Reshape  OutputDimensionality=Row vector (2-D)
  AoA/Beta : Subsystem
  Body Frame F & M : Subsystem
  Bus Creator : BusCreator  Inputs=2
  Bus Selector1 : BusSelector  OutputSignals=Fb,Mb
  Bus Selector2 : BusSelector  OutputSignals=aoa,beta
  Math Function1 : Math  Operator=transpose  SignedPower=on
  Reshape : Reshape  OutputDimensionality=Column vector (2-D)
  Sum2 : Sum  Inputs=|++  SaturateOnIntegerOverflow=on
  U2B1 : Subsystem
  U2B2 : Subsystem
  Vair : Sum  Inputs=+-  InputSameDT=on  SaturateOnIntegerOverflow=on  OutDataTypeStr=Inherit: Same as first input
  Weight matrix : Constant  Value=[0 0 mass*ISA_g]  VectorParams1D=off
  F&M b : Outport
  VT : Outport  Port=2
  tag scope: Vbcorrected=global, qS=global
  wires:
  Wind_e/1 -> Vair/2
  Ve/1 -> Vair/1
  Vair/1 -> 1xD/1
  U2B2/1(Out) -> AoA/Beta/1(Vb), Math Function1/1  "Vb"
  Weight matrix/1 -> U2B1/2(Vector 1x3)
  Den/1 -> AoA/Beta/2(den)
  Body Frame F & M/1(F&M_b) -> Bus Selector1/1
  Bus Selector1/1 -> 1 xD/1  "<Fb>"
  Bus Selector1/2 -> 1x D/1  "<Mb>"
  1xD/1 -> U2B2/1(Vector 1x3)
  1 xD/1 -> Sum2/1
  U2B1/1(Out) -> Sum2/2  "Fpl_b"
  Bus Creator/1 -> Reshape/1
  AoA/Beta/2(qS) -> [qS]
  Reshape/1 -> F&M b/1
  Euler/1 -> U2B2/2(roll/pitch/yaw), U2B1/1(roll/pitch/yaw)
  Math Function1/1 -> [Vbcorrected]
  Bus Selector2/2 -> Body Frame F & M/2("Beta, deg")  "<beta>"
  Bus Selector2/1 -> Body Frame F & M/1("Alpha, deg")  "<aoa>"
  da/1 -> Body Frame F & M/4("Da, deg")
  dr/1 -> Body Frame F & M/5("Dr, deg")
  de/1 -> Body Frame F & M/3("De, deg")
  1x D/1 -> Bus Creator/2  "Mb"
  Sum2/1 -> Bus Creator/1  "Fb"
  AoA/Beta/1("aoa/beta, deg") -> Bus Selector2/1
  AoA/Beta/3(VT) -> VT/1

== system sixdof/A//C/Global PQR ==
  In1 : Inport
  Selector : Selector  InputPortWidth=3  IndexOptions=Index vector (dialog)  Indices=[2]  OutputSizes=1
  Selector1 : Selector  InputPortWidth=3  IndexOptions=Index vector (dialog)  Indices=[1]  OutputSizes=1
  Selector2 : Selector  InputPortWidth=3  IndexOptions=Index vector (dialog)  Indices=[3]  OutputSizes=1
  tag scope: p=global, q=global, r=global
  wires:
  Selector/1 -> [q]
  In1/1 -> Selector/1, Selector1/1, Selector2/1
  Selector1/1 -> [p]
  Selector2/1 -> [r]

== system sixdof/A//C/ISA Atmosphere & Winds ==
  Pos_e : Inport
  ISA : Subsystem  mask(International Standart Atmosphere){L=ISA_lapse, h_lim=ISA_hmax, R=ISA_R, g=ISA_g, rh0=ISA_rho0, P0=ISA_P0, T0=ISA_T0}
      mask prompts: L "Lapse rate"; h_lim "Upper altitude limit, (m)"; R "Universal gas constant R"; g "Garvity constant, (m/c^2)"; rh0 "Sea level density, (kg/m^3)"; P0 "Sea level pressure, (N/m^2)"; T0 "Sea level temperature, (K)"
  Selector : Selector  InputPortWidth=3  IndexOptions=Index vector (dialog)  Indices=[3]  OutputSizes=1
  Terminator : Terminator
  Terminator1 : Terminator
  Terminator2 : Terminator
  Wind model : Subsystem
  Den : Outport
  Wind : Outport  Port=2
  wires:
  Pos_e/1 -> Selector/1
  Selector/1 -> ISA/1(height (m)), Wind model/1("Alt, m")
  ISA/4(Air Density (Kg/m^3)) -> Den/1
  ISA/1(Temperature (K)) -> Terminator/1
  ISA/2("Speed of Sound (m/s) ") -> Terminator1/1
  ISA/3("Air Pressure (N/m^2) ") -> Terminator2/1
  Wind model/1(Wind) -> Wind/1

== system sixdof/A//C/Output ==
  Mux : Mux  Inputs=7
  R2D : Gain  Gain=180/pi  SaturateOnIntegerOverflow=on  OutDataTypeStr=Inherit: Same as input  ParamDataTypeStr=Inherit: Same as input
  To File : ToFile  Filename=simout.mat  MatrixName=simout
  wires:
  [pqr] -> Mux/6
  [Ve] -> Mux/5
  [Pe] -> Mux/4
  [Vb] -> Mux/3
  [Controls] -> Mux/1
  Mux/1 -> To File/1
  R2D/1 -> Mux/7
  [aoa_beta] -> Mux/2
  [Euler] -> R2D/1

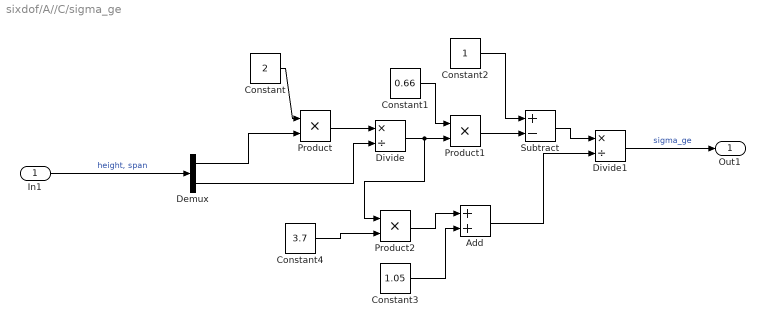
== system sixdof/A//C/sigma_ge ==
  In1 : Inport
  Add : Sum
  Constant : Constant  Value=2
  Constant1 : Constant  Value=0.66
  Constant2 : Constant
  Constant3 : Constant  Value=1.05
  Constant4 : Constant  Value=3.7
  Demux : Demux  Outputs=2
  Divide : Product  Inputs=*/
  Divide1 : Product  Inputs=*/
  Product : Product
  Product1 : Product
  Product2 : Product
  Subtract : Sum  Inputs=+-
  Out1 : Outport
  wires:
  In1/1 -> Demux/1  "height, span"
  Constant/1 -> Product/1
  Demux/1 -> Product/2
  Product/1 -> Divide/1
  Demux/2 -> Divide/2
  Divide/1 -> Product2/1, Product1/2
  Constant1/1 -> Product1/1
  Constant2/1 -> Subtract/1
  Product1/1 -> Subtract/2
  Subtract/1 -> Divide1/1
  Constant4/1 -> Product2/2
  Product2/1 -> Add/1
  Constant3/1 -> Add/2
  Add/1 -> Divide1/2
  Divide1/1 -> Out1/1  "sigma_ge"

== system sixdof/A//C/6DoF EoM/Direction Cosine Matrix from Euler Angles ==
  phi theta psi : Inport
  11 : Fcn  Expr=cos(u[3])*cos(u[2])
  12 : Fcn  Expr=sin(u[3])*cos(u[2])
  13 : Fcn  Expr=-sin(u[2])
  21 : Fcn  Expr=cos(u[3])*sin(u[2])*sin(u[1])-sin(u[3])*cos(u[1])
  22 : Fcn  Expr=sin(u[3])*sin(u[2])*sin(u[1])+cos(u[3])*cos(u[1])
  23 : Fcn  Expr=cos(u[2])*sin(u[1])
  31 : Fcn  Expr=cos(u[3])*sin(u[2])*cos(u[1])+sin(u[3])*sin(u[1])
  32 : Fcn  Expr=sin(u[3])*sin(u[2])*cos(u[1])-cos(u[3])*sin(u[1])
  33 : Fcn  Expr=cos(u[2])*cos(u[1])
  Mux2 : Mux  Inputs=9
  DCM : Outport  InitialOutput=0
  wires:
  33/1 -> Mux2/9
  32/1 -> Mux2/8
  31/1 -> Mux2/7
  23/1 -> Mux2/6
  22/1 -> Mux2/5
  21/1 -> Mux2/4
  13/1 -> Mux2/3
  12/1 -> Mux2/2
  11/1 -> Mux2/1
  Mux2/1 -> DCM/1
  phi theta psi/1 -> 11/1, 33/1, 32/1, 31/1, 23/1, 22/1, 21/1, 13/1, 12/1

== system sixdof/A//C/6DoF EoM/[V1,2,3,W1,2,3] ==
  note: V*dot =Inv(A){[F ; M] - SigmaAV*}
  "[F ; M]" : Inport
  V* : Inport  Port=2  PortDimensions=6
  A Matrix : Subsystem
  Demux : Demux  Outputs=[3;3]
      settings: DisplayOption=none
  Sigma : Subsystem
  Sigma*A : Product  Multiplication=Matrix(*)  InputSameDT=on  SaturateOnIntegerOverflow=on  OutDataTypeStr=Inherit: Same as first input
  Sigma*A*V* : Product  Multiplication=Matrix(*)  InputSameDT=on  SaturateOnIntegerOverflow=on  OutDataTypeStr=Inherit: Same as first input
  Sum1 : Sum  Inputs=+-|  InputSameDT=on  SaturateOnIntegerOverflow=on  OutDataTypeStr=Inherit: Same as first input
  Terminator1 : Terminator
  "V*dot " : Product  Inputs=/*  Multiplication=Matrix(*)  InputSameDT=on  SaturateOnIntegerOverflow=on  OutDataTypeStr=Inherit: Same as first input
  V*dot : Outport
  wires:
  Sigma*A/1 -> Sigma*A*V*/1
  "V*dot "/1 -> V*dot/1
  V*/1 -> Demux/1, Sigma*A*V*/2
  Demux/2 -> Sigma/1(pqr)
  Sigma*A*V*/1 -> Sum1/2
  "[F ; M]"/1 -> Sum1/1
  Sigma/1(Sigma) -> Sigma*A/1
  Demux/1 -> Terminator1/1
  A Matrix/1(A Matrix) -> Sigma*A/2, "V*dot "/1
  Sum1/1 -> "V*dot "/2

== system sixdof/A//C/6DoF EoM/phidot thetadot psidot ==
  p q r : Inport
  phi theta psi : Inport  Port=2
  Mux1 : Mux  Inputs=[3 3]
  Mux2 : Mux  Inputs=3
  phidot : Fcn  Expr=u[1]+u[2]*sin(u[4])*tan(u[5])+u[3]*cos(u[4])*tan(u[5])
  psidot : Fcn  Expr=u[2]*sin(u[4])/cos(u[5])+u[3]*cos(u[4])/cos(u[5])
  thetadot : Fcn  Expr=u[2]*cos(u[4])-u[3]*sin(u[4])
  phidot thetadot psidot : Outport  InitialOutput=0
  wires:
  Mux2/1 -> phidot thetadot psidot/1
  phidot/1 -> Mux2/1
  thetadot/1 -> Mux2/2
  psidot/1 -> Mux2/3
  phi theta psi/1 -> Mux1/2
  p q r/1 -> Mux1/1
  Mux1/1 -> thetadot/1, phidot/1, psidot/1

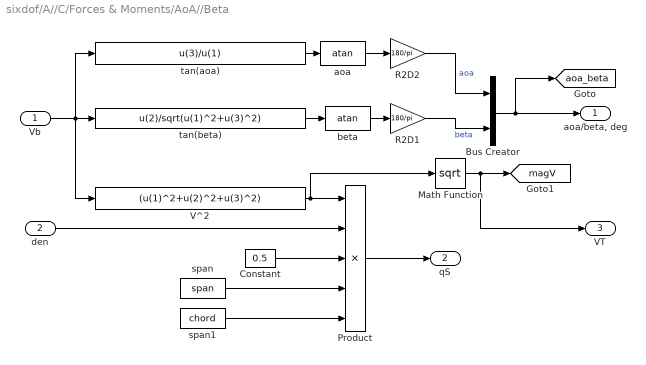
== system sixdof/A//C/Forces & Moments/AoA//Beta ==
  Vb : Inport
  den : Inport  Port=2
  Bus Creator : BusCreator  Inputs=2
  Constant : Constant  Value=0.5  VectorParams1D=off
  Math Function : Math  Operator=sqrt  SignedPower=on
  Product : Product  Inputs=5  SaturateOnIntegerOverflow=on  OutDataTypeStr=Inherit: Same as first input
  R2D1 : Gain  Gain=180/pi  SaturateOnIntegerOverflow=on  OutDataTypeStr=Inherit: Same as input  ParamDataTypeStr=Inherit: Same as input
  R2D2 : Gain  Gain=180/pi  SaturateOnIntegerOverflow=on  OutDataTypeStr=Inherit: Same as input  ParamDataTypeStr=Inherit: Same as input
  V^2 : Fcn  Expr=(u(1)^2+u(2)^2+u(3)^2)
  aoa : Trigonometry  Operator=atan
  beta : Trigonometry  Operator=atan
  span : Constant  Value=span  VectorParams1D=off
  span1 : Constant  Value=chord  VectorParams1D=off
  tan(aoa) : Fcn  Expr=u(3)/u(1)
  tan(beta) : Fcn  Expr=u(2)/sqrt(u(1)^2+u(3)^2)
  "aoa/beta, deg" : Outport
  qS : Outport  Port=2
  VT : Outport  Port=3
  tag scope: aoa_beta=global, magV=global
  wires:
  Vb/1 -> tan(beta)/1, V^2/1, tan(aoa)/1
  tan(beta)/1 -> beta/1
  beta/1 -> R2D1/1
  V^2/1 -> Product/1, Math Function/1
  den/1 -> Product/2
  Constant/1 -> Product/3
  Product/1 -> qS/1
  span/1 -> Product/4
  span1/1 -> Product/5
  R2D1/1 -> Bus Creator/2  "beta"
  aoa/1 -> R2D2/1
  R2D2/1 -> Bus Creator/1  "aoa"
  tan(aoa)/1 -> aoa/1
  Math Function/1 -> [magV], VT/1
  Bus Creator/1 -> "aoa/beta, deg"/1, [aoa_beta]

== system sixdof/A//C/Forces & Moments/Body Frame F & M ==
  "Alpha, deg" : Inport
  "Beta, deg" : Inport  Port=2
  "De, deg" : Inport  Port=3
  "Da, deg" : Inport  Port=4
  "Dr, deg" : Inport  Port=5
  Bus Creator : BusCreator  Inputs=2
  Transfer to body frame : Subsystem
  Wind frame F& M : Subsystem
  F&M_b : Outport
  wires:
  "Alpha, deg"/1 -> Wind frame F& M/1("Alpha, deg"), Bus Creator/1
  "Beta, deg"/1 -> Wind frame F& M/2("Beta, deg"), Bus Creator/2
  "Dr, deg"/1 -> Wind frame F& M/5("Dr, deg")
  "Da, deg"/1 -> Wind frame F& M/4("Da, deg")
  "De, deg"/1 -> Wind frame F& M/3("De, deg")
  Wind frame F& M/1(F&M wind frame) -> Transfer to body frame/1(Wind frame F&M)
  Bus Creator/1 -> Transfer to body frame/2("aoa/beta, deg")  "aoa/beta, deg"
  Transfer to body frame/1(F&M_b) -> F&M_b/1

== system sixdof/A//C/Forces & Moments/U2B1 ==
  roll/pitch/yaw : Inport
  Vector 1x3 : Inport  Port=2
  Math Function : Math  Operator=transpose  SignedPower=on
  Product1 : Product  Multiplication=Matrix(*)  InputSameDT=on  SaturateOnIntegerOverflow=on  OutDataTypeStr=Inherit: Same as first input
  Rb2u : Subsystem
  Reshape : Reshape  OutputDimensionality=Column vector (2-D)
  Reshape1 : Reshape  OutputDimensionality=Row vector (2-D)
  Out : Outport
  wires:
  Rb2u/1(DCM) -> Math Function/1
  roll/pitch/yaw/1 -> Rb2u/1(phi theta psi)
  Product1/1 -> Reshape1/1
  Math Function/1 -> Product1/1
  Vector 1x3/1 -> Reshape/1
  Reshape1/1 -> Out/1
  Reshape/1 -> Product1/2

== system sixdof/A//C/Forces & Moments/U2B2 ==
  Vector 1x3 : Inport
  roll/pitch/yaw : Inport  Port=2
  Math Function : Math  Operator=transpose  SignedPower=on
  Product1 : Product  Multiplication=Matrix(*)  InputSameDT=on  SaturateOnIntegerOverflow=on  OutDataTypeStr=Inherit: Same as first input
  Rb2u : Subsystem
  Reshape : Reshape  OutputDimensionality=Column vector (2-D)
  Reshape1 : Reshape  OutputDimensionality=Row vector (2-D)
  Out : Outport
  wires:
  Product1/1 -> Reshape1/1
  roll/pitch/yaw/1 -> Rb2u/1(phi theta psi)
  Rb2u/1(DCM) -> Math Function/1
  Math Function/1 -> Product1/1
  Vector 1x3/1 -> Reshape/1
  Reshape/1 -> Product1/2
  Reshape1/1 -> Out/1

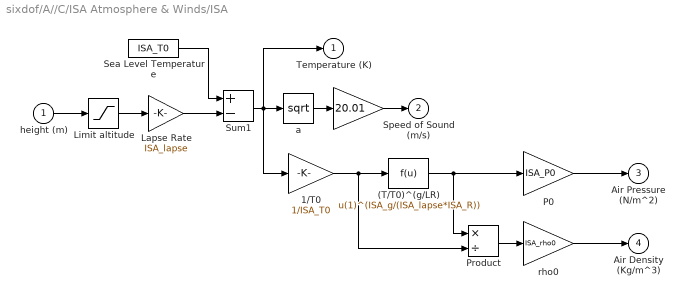
== system sixdof/A//C/ISA Atmosphere & Winds/ISA ==
  height (m) : Inport
  " " : Gain  Gain=20.01  SaturateOnIntegerOverflow=on  OutDataTypeStr=Inherit: Same as input  ParamDataTypeStr=Inherit: Same as input
  (T/T0)^(g/LR) : Fcn  Expr=u(1)^(ISA_g/(ISA_lapse*ISA_R))
  1/T0 : Gain  Gain=1/ISA_T0  SaturateOnIntegerOverflow=on  OutDataTypeStr=Inherit: Same as input  ParamDataTypeStr=Inherit: Same as input
  Lapse Rate : Gain  Gain=ISA_lapse  SaturateOnIntegerOverflow=on  OutDataTypeStr=Inherit: Same as input  ParamDataTypeStr=Inherit: Same as input
  Limit altitude : Saturate  UpperLimit=ISA_hmax  LowerLimit=0
  P0 : Gain  Gain=ISA_P0  SaturateOnIntegerOverflow=on  OutDataTypeStr=Inherit: Same as input  ParamDataTypeStr=Inherit: Same as input
  Product : Product  Inputs=*/  InputSameDT=on  SaturateOnIntegerOverflow=on  OutDataTypeStr=Inherit: Same as first input
  Sea Level Temperature : Constant  Value=ISA_T0
  Sum1 : Sum  Inputs=+-  InputSameDT=on  SaturateOnIntegerOverflow=on  OutDataTypeStr=Inherit: Same as first input
  a : Math  Operator=sqrt  SignedPower=on
  rho0 : Gain  Gain=ISA_rho0  SaturateOnIntegerOverflow=on  OutDataTypeStr=Inherit: Same as input  ParamDataTypeStr=Inherit: Same as input
  Temperature (K) : Outport  InitialOutput=0
  "Speed of Sound (m/s) " : Outport  Port=2  InitialOutput=0
  "Air Pressure (N/m^2) " : Outport  Port=3  InitialOutput=0
  Air Density (Kg/m^3) : Outport  Port=4  InitialOutput=0
  wires:
  rho0/1 -> Air Density (Kg/m^3)/1
  P0/1 -> "Air Pressure (N/m^2) "/1
  Sea Level Temperature/1 -> Sum1/1
  Sum1/1 -> a/1, Temperature (K)/1, 1/T0/1
  1/T0/1 -> (T/T0)^(g/LR)/1, Product/2
  (T/T0)^(g/LR)/1 -> P0/1, Product/1
  Product/1 -> rho0/1
  Limit altitude/1 -> Lapse Rate/1
  height (m)/1 -> Limit altitude/1
  a/1 -> " "/1
  " "/1 -> "Speed of Sound (m/s) "/1
  Lapse Rate/1 -> Sum1/2

== system sixdof/A//C/ISA Atmosphere & Winds/Wind model ==
  "Alt, m" : Inport
  GetWind : Subsystem
  Matrix Gain6 : Gain  Gain="[1 0 0 ;0 1 0 ;0  0 -1]"  Multiplication=Matrix(K*u)  SaturateOnIntegerOverflow=on  OutDataTypeStr=Inherit: Same as input  ParamDataTypeStr=Inherit: Same as input
  Reshape : Reshape  OutputDimensionality=Customize  OutputDimensions=[3,1]
  Wind : Outport
  wires:
  GetWind/1(WindOut) -> Matrix Gain6/1
  Matrix Gain6/1 -> Reshape/1
  Reshape/1 -> Wind/1
  "Alt, m"/1 -> GetWind/1(Alt)

== system sixdof/A//C/6DoF EoM/[V1,2,3,W1,2,3]/A Matrix ==
  Constant1 : Constant  Value=zeros(3,3)
  Constant4 : Constant  Value=0
  Ixx : Constant  Value=Ixx  VectorParams1D=off
  Iyy : Constant  Value=Iyy  VectorParams1D=off
  Izz : Constant  Value=Izz  VectorParams1D=off
  Matrix Concatenation : Concatenate  Mode=Multidimensional array
  Matrix Concatenation1 : Concatenate  Mode=Multidimensional array
  Matrix Concatenation2 : Concatenate  Mode=Multidimensional array  ConcatenateDimension=2
  Mux : Mux  Inputs=9
  Mux1 : Mux  Inputs=9
  Reshape : Reshape  OutputDimensionality=Customize  OutputDimensions=[3,3]
  Reshape1 : Reshape  OutputDimensionality=Customize  OutputDimensions=[3,3]
  mass : Constant  Value=mass  VectorParams1D=off
  A Matrix : Outport
  wires:
  Ixx/1 -> Mux/1
  Izz/1 -> Mux/9
  Iyy/1 -> Mux/5
  Constant4/1 -> Mux/8, Mux/7, Mux/6, Mux/4, Mux/3, Mux/2, Mux1/8, Mux1/7, Mux1/6, Mux1/4, Mux1/3, Mux1/2
  mass/1 -> Mux1/1, Mux1/5, Mux1/9
  Mux1/1 -> Reshape/1
  Mux/1 -> Reshape1/1
  Matrix Concatenation/1 -> Matrix Concatenation2/1
  Matrix Concatenation1/1 -> Matrix Concatenation2/2
  Matrix Concatenation2/1 -> A Matrix/1
  Reshape1/1 -> Matrix Concatenation1/2
  Reshape/1 -> Matrix Concatenation/1
  Constant1/1 -> Matrix Concatenation/2, Matrix Concatenation1/1

== system sixdof/A//C/6DoF EoM/[V1,2,3,W1,2,3]/Sigma ==
  note: S(pqr)
  pqr : Inport
  Gain : Gain  Gain=[0 0 0;0 0 -1; 0 1 0]  Multiplication=Matrix(K*u)  SaturateOnIntegerOverflow=on  OutDataTypeStr=Inherit: Same as input  ParamDataTypeStr=Inherit: Same as input
  Gain1 : Gain  Gain=[0 0 1;0 0 0; -1 0 0]  Multiplication=Matrix(K*u)  SaturateOnIntegerOverflow=on  OutDataTypeStr=Inherit: Same as input  ParamDataTypeStr=Inherit: Same as input
  Gain2 : Gain  Gain="[0 -1 0;1 0 0;  0 0 0]"  Multiplication=Matrix(K*u)  SaturateOnIntegerOverflow=on  OutDataTypeStr=Inherit: Same as input  ParamDataTypeStr=Inherit: Same as input
  Gain3 : Gain  Gain=0  SaturateOnIntegerOverflow=on  OutDataTypeStr=Inherit: Same as input  ParamDataTypeStr=Inherit: Same as input
  Math Function : Math  Operator=transpose  SignedPower=on
  Matrix Concatenation : Concatenate  Mode=Multidimensional array  ConcatenateDimension=2
  Matrix Concatenation1 : Concatenate  Mode=Multidimensional array  ConcatenateDimension=2
  Matrix Concatenation2 : Concatenate  Mode=Multidimensional array
  Mux : Mux  Inputs=3
  Reshape : Reshape  OutputDimensionality=Customize  OutputDimensions=[3,3]
  Sigma : Outport
  wires:
  Mux/1 -> Reshape/1
  Gain/1 -> Mux/1
  Gain1/1 -> Mux/2
  Gain2/1 -> Mux/3
  Reshape/1 -> Math Function/1
  Math Function/1 -> Gain3/1, Matrix Concatenation/1, Matrix Concatenation1/2
  Gain3/1 -> Matrix Concatenation/2, Matrix Concatenation1/1
  Matrix Concatenation/1 -> Matrix Concatenation2/1
  Matrix Concatenation1/1 -> Matrix Concatenation2/2
  Matrix Concatenation2/1 -> Sigma/1
  pqr/1 -> Gain/1, Gain1/1, Gain2/1

== system sixdof/A//C/Forces & Moments/Body Frame F & M/Transfer to body frame ==
  Wind frame F&M : Inport
  "aoa/beta, deg" : Inport  Port=2
  Bus Creator1 : BusCreator  Inputs=2
  D2R : Gain  Gain=pi/180  SaturateOnIntegerOverflow=on  OutDataTypeStr=Inherit: Same as input  ParamDataTypeStr=Inherit: Same as input
  Forces : Selector  InputPortWidth=6  IndexOptions=Index vector (dialog)  Indices=[1 2 3]  OutputSizes=1
  Moments : Selector  InputPortWidth=6  IndexOptions=Index vector (dialog)  Indices=[4 5 6]  OutputSizes=1
  Ra2b1 : Subsystem
  Ra2b22 : Subsystem
  F&M_b : Outport
  wires:
  Ra2b1/1(body frame) -> Bus Creator1/1  "Fb"
  Ra2b22/1(body frame) -> Bus Creator1/2  "Mb"
  "aoa/beta, deg"/1 -> D2R/1
  Forces/1 -> Ra2b1/1(wind frame)
  Wind frame F&M/1 -> Forces/1, Moments/1
  Bus Creator1/1 -> F&M_b/1
  Moments/1 -> Ra2b22/2(wind frame)
  D2R/1 -> Ra2b1/2(aoa/beta), Ra2b22/1(aoa/beta)
